simulink library "ProductionLinePLib"  (R2025a)
settings: Solver=VariableStepAuto  StartTime=0.0  StopTime=10.0  RelTol=1e-3
libraries: StdLib x118, $bdroot x44
(part 2 of 2)

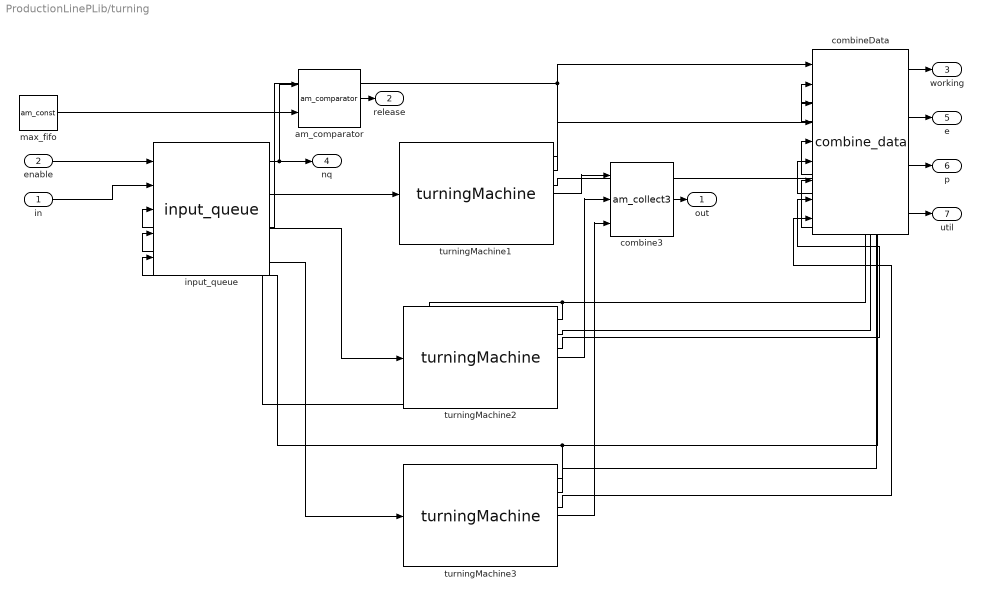
== system ProductionLinePLib/turning ==
  in : Inport
  enable : Inport  Port=2
  am_comparator : StdLib/am_comparator  compop="\"<\""  tau=[0,1]  debug=0
      settings: SourceProductName=Math Operations
  combine3 : StdLib/am_collect3  tD=[0,10]  tau=[0,1]  debug=debug
      settings: SourceProductName=Routing
  combineData : $bdroot/combine_data  tau=[0,1]  debug=0
  input_queue : $bdroot/input_queue  tD=[0,5]  tau=[0,5]  debug=debug
  max_fifo : StdLib/am_const  value=max_fifo  sendTime=[0,1]  debug=debug
      settings: SourceProductName=Sources
  turningMachine1 : $bdroot/turningMachine  turning_time=20*60  ap_ug=0.5  ap_og=1.5  P_ap=0.6  f_ug=0.1  f_og=0.5  P_f=0.4  vc_ug=150  vc_og=350  P_vc=0.5  ap=ap  f=f  vc=vc  tauInt=tauInt  tauCont=tauCont  tau=[0,1]  debug=debug
  turningMachine2 : $bdroot/turningMachine  turning_time=20*60  ap_ug=0.5  ap_og=1.5  P_ap=0.6  f_ug=0.1  f_og=0.5  P_f=0.4  vc_ug=150  vc_og=350  P_vc=0.5  ap=ap  f=f  vc=vc  tauInt=tauInt  tauCont=tauCont  tau=[0,1]  debug=debug
  turningMachine3 : $bdroot/turningMachine  turning_time=20*60  ap_ug=0.5  ap_og=1.5  P_ap=0.6  f_ug=0.1  f_og=0.5  P_f=0.4  vc_ug=150  vc_og=350  P_vc=0.5  ap=ap  f=f  vc=vc  tauInt=tauInt  tauCont=tauCont  tau=[0,1]  debug=debug
  out : Outport
  release : Outport  Port=2
  working : Outport  Port=3
  nq : Outport  Port=4
  e : Outport  Port=5
  p : Outport  Port=6
  util : Outport  Port=7
  wires:
  turningMachine2/2 -> combineData/2, input_queue/4
  turningMachine1/2 -> combineData/1, input_queue/3
  turningMachine1/1 -> combine3/1
  turningMachine2/1 -> combine3/2
  turningMachine3/1 -> combine3/3
  combine3/1 -> out/1
  turningMachine3/2 -> combineData/3, input_queue/5
  enable/1 -> input_queue/1
  in/1 -> input_queue/2
  input_queue/1 -> am_comparator/1, nq/1
  input_queue/2 -> turningMachine1/1
  input_queue/3 -> turningMachine2/1
  input_queue/4 -> turningMachine3/1
  turningMachine1/3 -> combineData/4
  turningMachine1/4 -> combineData/7
  turningMachine2/3 -> combineData/5
  turningMachine2/4 -> combineData/8
  turningMachine3/3 -> combineData/6
  turningMachine3/4 -> combineData/9
  combineData/1 -> working/1
  combineData/3 -> p/1
  combineData/2 -> e/1
  combineData/4 -> util/1
  am_comparator/1 -> release/1
  max_fifo/1 -> am_comparator/2

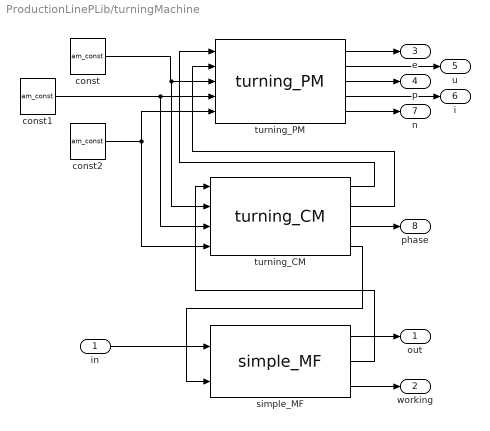
== system ProductionLinePLib/turningMachine ==
  in : Inport
  const : StdLib/am_const  value=ap  sendTime=[0,1]  debug=0
      settings: SourceProductName=Sources
  const1 : StdLib/am_const  value=f  sendTime=[0,1]  debug=0
      settings: SourceProductName=Sources
  const2 : StdLib/am_const  value=vc  sendTime=[0,1]  debug=0
      settings: SourceProductName=Sources
  simple_MF : $bdroot/simple_MF  tau=tau  debug=debug
  turning_CM : $bdroot/turning_CM  turning_time=turning_time  ap_ug=ap_ug  f_ug=f_ug  vc_ug=vc_ug  ap_og=ap_og  f_og=f_og  vc_og=vc_og  tau=tauCont  debug=debug
  turning_PM : $bdroot/turning_PM  R=6  L=0.2  J=0.052  b=0.015  K=0.15  vcc=150  vcc_load=30  load=0.75/200  ap_ug=ap_ug  f_ug=f_ug  vc_ug=vc_ug  ap_og=ap_og  f_og=f_og  vc_og=vc_og  P_ap=P_ap  P_f=P_f  P_vc=P_vc  tauInt=tauInt  tau=tau  debug=debug
  out : Outport
  working : Outport  Port=2
  e : Outport  Port=3
  p : Outport  Port=4
  u : Outport  Port=5
  i : Outport  Port=6
  n : Outport  Port=7
  phase : Outport  Port=8
  wires:
  simple_MF/2 -> turning_CM/1
  turning_CM/4 -> simple_MF/2
  turning_CM/2 -> turning_PM/2
  turning_CM/1 -> turning_PM/1
  turning_PM/3 -> p/1
  turning_PM/1 -> e/1
  simple_MF/3 -> working/1
  simple_MF/1 -> out/1
  in/1 -> simple_MF/1
  turning_PM/2 -> u/1
  turning_PM/4 -> i/1
  turning_PM/5 -> n/1
  turning_CM/3 -> phase/1
  const1/1 -> turning_CM/3, turning_PM/4
  const2/1 -> turning_PM/5, turning_CM/4
  const/1 -> turning_CM/2, turning_PM/3

== system ProductionLinePLib/turningMotorI ==
  u : Inport
  n : Inport  Port=2
  add3 : StdLib/am_add3  tau=tau  debug=debug
      settings: SourceProductName=Math Operations
  gain : StdLib/am_gain  g=1/L  tau=[0,1]  debug=debug
      settings: SourceProductName=Math Operations
  gain1 : StdLib/am_gain  g=-K  tau=tau  debug=debug
      settings: SourceProductName=Math Operations
  gain2 : StdLib/am_gain  g=-R  tau=[0,1]  debug=debug
      settings: SourceProductName=Math Operations
  hIntegrator : StdLib/am_hIntegrator  dq=5  epsilon=100  X0=0  tau=tauInt  debug=debug
      settings: SourceProductName=QSS
  i : Outport
  wires:
  n/1 -> gain1/1
  add3/1 -> gain/1
  gain/1 -> hIntegrator/1
  gain1/1 -> add3/3
  hIntegrator/1 -> gain2/1, i/1
  u/1 -> add3/2
  gain2/1 -> add3/1

== system ProductionLinePLib/turningMotorN ==
  i : Inport
  turning : Inport  Port=2
  add3 : StdLib/am_add3  tau=[0,1]  debug=debug
      settings: SourceProductName=Math Operations
  const : StdLib/am_const  value=load  sendTime=[0,1]  debug=debug
      settings: SourceProductName=Sources
  gain : StdLib/am_gain  g=-1  tau=[0,1]  debug=debug
      settings: SourceProductName=Math Operations
  gain1 : StdLib/am_gain  g=K  tau=tau  debug=debug
      settings: SourceProductName=Math Operations
  gain2 : StdLib/am_gain  g=1/J  tau=[0,1]  debug=debug
      settings: SourceProductName=Math Operations
  gain3 : StdLib/am_gain  g=30/pi  tau=[0,1]  debug=debug
      settings: SourceProductName=Math Operations
  gain4 : StdLib/am_gain  g=-b  tau=[0,1]  debug=debug
      settings: SourceProductName=Math Operations
  hIntegrator : StdLib/am_hIntegrator  dq=50  epsilon=100  X0=0  tau=tauInt  debug=debug
      settings: SourceProductName=QSS
  mult3 : StdLib/am_mult3  tau=tau  debug=debug
      settings: SourceProductName=Math Operations
  n : Outport
  n_rad : Outport  Port=2
  wires:
  add3/1 -> gain2/1
  turning/1 -> mult3/2
  const/1 -> mult3/1
  mult3/1 -> gain/1
  gain4/1 -> add3/3
  hIntegrator/1 -> gain3/1, gain4/1, mult3/3, n_rad/1
  gain3/1 -> n/1
  gain2/1 -> hIntegrator/1
  gain/1 -> add3/2
  i/1 -> gain1/1
  gain1/1 -> add3/1

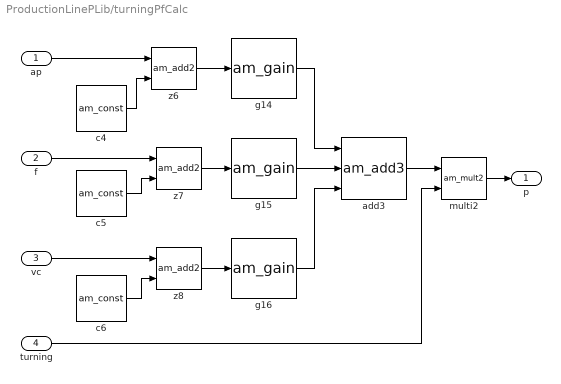
== system ProductionLinePLib/turningPfCalc ==
  ap : Inport
  f : Inport  Port=2
  vc : Inport  Port=3
  turning : Inport  Port=4
  add3 : StdLib/am_add3  tau=[0,1]  debug=debug
      settings: SourceProductName=Math Operations
  c4 : StdLib/am_const  value=-ap_ug  sendTime=[0,1]  debug=debug
      settings: SourceProductName=Sources
  c5 : StdLib/am_const  value=-f_ug  sendTime=[0,1]  debug=debug
      settings: SourceProductName=Sources
  c6 : StdLib/am_const  value=-vc_ug  sendTime=[0,1]  debug=debug
      settings: SourceProductName=Sources
  g14 : StdLib/am_gain  g=1/(ap_og - ap_ug)*P_ap  tau=[0,1]  debug=debug
      settings: SourceProductName=Math Operations
  g15 : StdLib/am_gain  g=1/(f_og - f_ug)*P_f  tau=[0,1]  debug=debug
      settings: SourceProductName=Math Operations
  g16 : StdLib/am_gain  g=1/(vc_og - vc_ug)*P_vc  tau=[0,1]  debug=debug
      settings: SourceProductName=Math Operations
  multi2 : StdLib/am_mult2  tau=tau  debug=debug
      settings: SourceProductName=Math Operations
  z6 : StdLib/am_add2  tau=tau  debug=debug
      settings: SourceProductName=Math Operations
  z7 : StdLib/am_add2  tau=tau  debug=debug
      settings: SourceProductName=Math Operations
  z8 : StdLib/am_add2  tau=tau  debug=debug
      settings: SourceProductName=Math Operations
  p : Outport
  wires:
  g14/1 -> add3/1
  g15/1 -> add3/2
  c6/1 -> z8/2
  z8/1 -> g16/1
  g16/1 -> add3/3
  turning/1 -> multi2/2
  z6/1 -> g14/1
  c4/1 -> z6/2
  z7/1 -> g15/1
  multi2/1 -> p/1
  c5/1 -> z7/2
  vc/1 -> z8/1
  add3/1 -> multi2/1
  ap/1 -> z6/1
  f/1 -> z7/1

== system ProductionLinePLib/turningPowerCalc ==
  p_in : Inport
  u_in : Inport  Port=2
  i_in : Inport  Port=3
  add2 : StdLib/am_add2  tau=tau  debug=debug
      settings: SourceProductName=Math Operations
  gain : StdLib/am_gain  g=1/1000  tau=[0,1]  debug=debug
      settings: SourceProductName=Math Operations
  gain1 : StdLib/am_gain  g=1/3600  tau=[0,1]  debug=debug
      settings: SourceProductName=Math Operations
  hIntegrator : StdLib/am_hIntegrator  dq=0.1  epsilon=0.2  X0=0  tau=tauInt  debug=debug
      settings: SourceProductName=QSS
  multi2 : StdLib/am_mult2  tau=tau  debug=debug
      settings: SourceProductName=Math Operations
  saturation : StdLib/am_saturation  ll=0  ul=Inf  tau=tau  debug=debug
      settings: SourceProductName=Math Operations
  i_out : Outport
  p_out : Outport  Port=2
  e_out : Outport  Port=3
  wires:
  multi2/1 -> gain/1
  saturation/1 -> multi2/1, i_out/1
  u_in/1 -> multi2/2
  i_in/1 -> saturation/1
  p_in/1 -> add2/1
  gain/1 -> add2/2
  add2/1 -> gain1/1, p_out/1
  hIntegrator/1 -> e_out/1
  gain1/1 -> hIntegrator/1

== system ProductionLinePLib/turningPowerSupply ==
  turning : Inport
  on : Inport  Port=2
  add2 : StdLib/am_add2  tau=[0,1]  debug=debug
      settings: SourceProductName=Math Operations
  const : StdLib/am_const  value=vcc_load  sendTime=[0,1]  debug=debug
      settings: SourceProductName=Sources
  const1 : StdLib/am_const  value=vcc  sendTime=[0,1]  debug=debug
      settings: SourceProductName=Sources
  multi1 : StdLib/am_mult2  tau=tau  debug=debug
      settings: SourceProductName=Math Operations
  multi2 : StdLib/am_mult2  tau=[0,1]  debug=debug
      settings: SourceProductName=Math Operations
  u : Outport
  wires:
  const1/1 -> add2/1
  turning/1 -> multi1/1
  const/1 -> multi1/2
  multi2/1 -> u/1
  on/1 -> multi2/2
  add2/1 -> multi2/1
  multi1/1 -> add2/2

== system ProductionLinePLib/turning_CM ==
  entered : Inport
  ap : Inport  Port=2
  f : Inport  Port=3
  vc : Inport  Port=4
  turning_controller1 : $bdroot/turning_controller  turning_time=turning_time  ap_ug=ap_ug  f_ug=f_ug  vc_ug=vc_ug  ap_og=ap_og  f_og=f_og  vc_og=vc_og  tau=tau  debug=debug
  on : Outport
  turning : Outport  Port=2
  phase : Outport  Port=3
  leaving : Outport  Port=4
  wires:
  vc/1 -> turning_controller1/4
  f/1 -> turning_controller1/3
  ap/1 -> turning_controller1/2
  turning_controller1/3 -> phase/1
  turning_controller1/2 -> turning/1
  turning_controller1/1 -> on/1
  entered/1 -> turning_controller1/1
  turning_controller1/4 -> leaving/1

== system ProductionLinePLib/turning_PM ==
  on : Inport
  turning : Inport  Port=2
  ap : Inport  Port=3
  f : Inport  Port=4
  vc : Inport  Port=5
  turningMotorI : $bdroot/turningMotorI  R=R  L=L  K=K  tauInt=tauInt  tau=[0,1]  debug=debug
  turningMotorN : $bdroot/turningMotorN  J=J  b=b  K=K  load=load  tauInt=tauInt  tau=[0,1]  debug=debug
  turningPfCalc : $bdroot/turningPfCalc  ap_ug=ap_ug  ap_og=ap_og  P_ap=P_ap  f_ug=f_ug  f_og=f_og  P_f=P_f  vc_ug=vc_ug  vc_og=vc_og  P_vc=P_vc  tau=tau  debug=debug
  turningPowerCalc : $bdroot/turningPowerCalc  tauInt=tauInt  tau=[0,1]  debug=debug
  turningPowerSupply : $bdroot/turningPowerSupply  vcc=vcc  vcc_load=vcc_load  tau=tau  debug=debug
  e : Outport
  u : Outport  Port=2
  p : Outport  Port=3
  i : Outport  Port=4
  n : Outport  Port=5
  wires:
  ap/1 -> turningPfCalc/1
  f/1 -> turningPfCalc/2
  vc/1 -> turningPfCalc/3
  turning/1 -> turningMotorN/2, turningPowerSupply/1, turningPfCalc/4
  turningPfCalc/1 -> turningPowerCalc/1
  turningPowerCalc/1 -> i/1
  turningPowerCalc/2 -> p/1
  turningPowerCalc/3 -> e/1
  turningMotorI/1 -> turningMotorN/1, turningPowerCalc/3
  turningMotorN/1 -> n/1
  turningMotorN/2 -> turningMotorI/2
  turningPowerSupply/1 -> turningMotorI/1, turningPowerCalc/2, u/1
  on/1 -> turningPowerSupply/2

== system ProductionLinePLib/turning_controller ==
  entered : Inport
  ap : Inport  Port=2
  f : Inport  Port=3
  vc : Inport  Port=4
  on : Outport
  turning : Outport  Port=2
  phase : Outport  Port=3
  leaving : Outport  Port=4
